simulink model "Challenge_integral"  (R2021a)
settings: Solver=VariableStepAuto  StartTime=0.0  StopTime=2.5  RelTol=1e-3
undefined symbols (not defined in the file): challint, degs2rpm, rpm2rads, sens
settings Model: Creator=gioel  LastModifiedBy=gioel

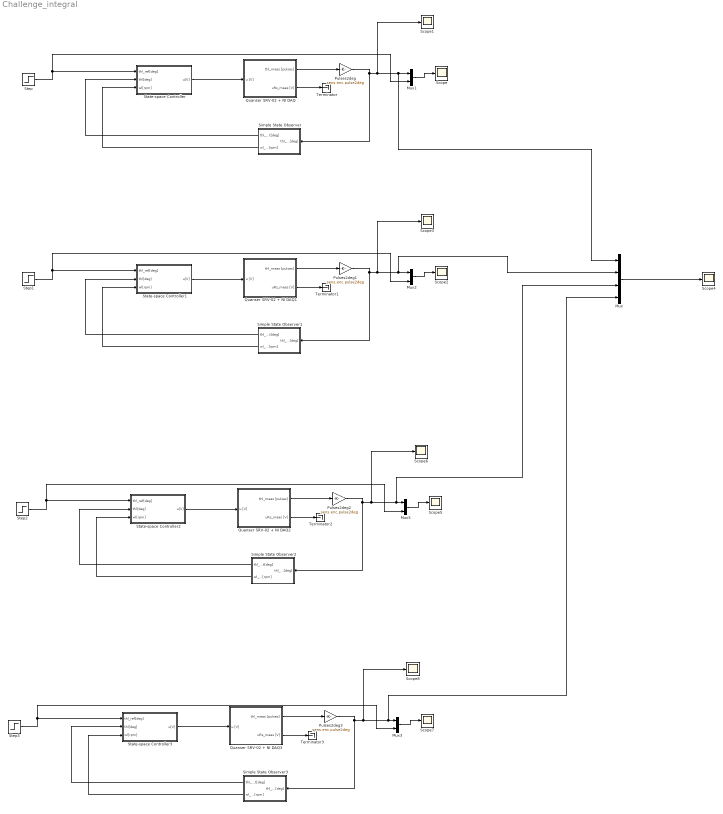
== system Challenge_integral ==
  Mux : Mux
  Mux{1..3,5} (4 alike) : Mux  Inputs=2
  Pulses2deg{,1..3} (4 alike) : Gain  Gain=sens.enc.pulse2deg
  Quanser SRV-02 + NI DAQ : Subsystem  mask(Quanser SRV-02 (with inertial load) + NI DAQ){Ts=0.001, fricType=Karnopp}
      mask prompts: Ts "NI DAQ Sample Time:"; fricType "Friction model"
      mask help: Quanser SRV-02 (with inertial load) + NI DAQ model.
      mask init:
      | %%  Sensors data
      | 
      | %   shunt resistor
      | sens.curr.Rs = 0.5;                         %   resistance [Ohm]   
      | sens.curr.uRs_std = 0.01;                   %   voltage noise standard dev [V]                           
      | sens.curr.uRs_var = sens.curr.uRs_std^2;	%   voltage noise variance [V^2]
      | 
      | %   Hewlett-Packard HEDS-5540#A06 optical encoder
      | sens.enc.ppr = 500*4;                       %   pulses per rotation
      | sens.enc.pulse2deg = 360/sens.enc.ppr;      %   [pulses] -> [deg]
      | sens.enc.pulse2rad = 2*pi/sens.enc.ppr;     %   [pulses] -> [rad]
      | sens.enc.deg2pulse = sens.enc.ppr/360;      %   [deg] -> [pulses]
      | sens.enc.rad2pulse = sens.enc.ppr/2/pi;     %   [rad] -> [pulses]
      | 
      | 
      | %%  Data acquisition board (daq) data
      | 
      | %   NI PCI-6221 DAC data
      | daq.dac.bits = 16;                                  %   resolution (bits)
      | daq.dac.fs   = 10;                                  %   full scale 
      | daq.dac.q    = 2*daq.dac.fs/(2^daq.dac.bits-1);     %	quantization
      | 
      | %   NI PCI-6221 ADC data
      | daq.adc.bits = 16;                                  %   resolution (bits)
      | daq.adc.fs   = 10;                                  %   full scale (as set in SLDRT Analog Input block)
      | daq.adc.q    = 2*daq.adc.fs/(2^daq.adc.bits-1);     %   quantization
      mask Help:
      | Riccardo Antonello (antonello@dei.unipd.it)
      | 
      | April 24, 2020
      | 
      | Dept. of Information Engineering, University of Padova
      mask TypeOptions fricType: Coulomb + viscous | Karnopp
  Quanser SRV-02 + NI DAQ1 : Subsystem  mask(Quanser SRV-02 (with inertial load) + NI DAQ){Ts=0.001, fricType=Karnopp}
      mask prompts: Ts "NI DAQ Sample Time:"; fricType "Friction model"
      mask help: Quanser SRV-02 (with inertial load) + NI DAQ model.
      mask init: same as Challenge_integral/Quanser SRV-02 + NI DAQ
      mask Help:
      | Riccardo Antonello (antonello@dei.unipd.it)
      | 
      | April 24, 2020
      | 
      | Dept. of Information Engineering, University of Padova
      mask TypeOptions fricType: Coulomb + viscous | Karnopp
  Quanser SRV-02 + NI DAQ2 : Subsystem  mask(Quanser SRV-02 (with inertial load) + NI DAQ){Ts=0.001, fricType=Karnopp}
      mask prompts: Ts "NI DAQ Sample Time:"; fricType "Friction model"
      mask help: Quanser SRV-02 (with inertial load) + NI DAQ model.
      mask init: same as Challenge_integral/Quanser SRV-02 + NI DAQ
      mask Help:
      | Riccardo Antonello (antonello@dei.unipd.it)
      | 
      | April 24, 2020
      | 
      | Dept. of Information Engineering, University of Padova
      mask TypeOptions fricType: Coulomb + viscous | Karnopp
  Quanser SRV-02 + NI DAQ3 : Subsystem  mask(Quanser SRV-02 (with inertial load) + NI DAQ){Ts=0.001, fricType=Karnopp}
      mask prompts: Ts "NI DAQ Sample Time:"; fricType "Friction model"
      mask help: Quanser SRV-02 (with inertial load) + NI DAQ model.
      mask init: same as Challenge_integral/Quanser SRV-02 + NI DAQ
      mask Help:
      | Riccardo Antonello (antonello@dei.unipd.it)
      | 
      | April 24, 2020
      | 
      | Dept. of Information Engineering, University of Padova
      mask TypeOptions fricType: Coulomb + viscous | Karnopp
  Scope{,1..8} (9 alike) : Scope
  Simple State Observer : Subsystem
  Simple State Observer1 : Subsystem
  Simple State Observer2 : Subsystem
  Simple State Observer3 : Subsystem
  State-space Controller : Subsystem
  State-space Controller1 : Subsystem
  State-space Controller2 : Subsystem
  State-space Controller3 : Subsystem
  Step{,1..3} (4 alike) : Step  Time=0  After=70  SampleTime=0
  Terminator{,1..3} (4 alike) : Terminator
  wires:
  Step/1 -> State-space Controller/1(thl_ref[deg]), Mux1/2
  Pulses2deg/1 -> Scope1/1, Mux/1, Mux1/1, Simple State Observer/1(thl_meas[deg])
  Mux1/1 -> Scope/1
  Quanser SRV-02 + NI DAQ/2(uRs_meas [V]) -> Terminator/1
  Quanser SRV-02 + NI DAQ/1(thl_meas [pulses]) -> Pulses2deg/1
  State-space Controller/1(u[V]) -> Quanser SRV-02 + NI DAQ/1(u [V])
  Simple State Observer/1(thl_est[deg]) -> State-space Controller/2(thl[deg])
  Simple State Observer/2(wl_est[rpm]) -> State-space Controller/3(wl[rpm])
  Step1/1 -> State-space Controller1/1(thl_ref[deg]), Mux2/2
  State-space Controller1/1(u[V]) -> Quanser SRV-02 + NI DAQ1/1(u [V])
  Pulses2deg1/1 -> Scope3/1, Mux/2, Mux2/1, Simple State Observer1/1(thl_meas[deg])
  Mux2/1 -> Scope2/1
  Quanser SRV-02 + NI DAQ1/2(uRs_meas [V]) -> Terminator1/1
  Simple State Observer1/2(wl_est[rpm]) -> State-space Controller1/3(wl[rpm])
  Simple State Observer1/1(thl_est[deg]) -> State-space Controller1/2(thl[deg])
  Quanser SRV-02 + NI DAQ1/1(thl_meas [pulses]) -> Pulses2deg1/1
  Step2/1 -> State-space Controller2/1(thl_ref[deg]), Mux5/2
  State-space Controller2/1(u[V]) -> Quanser SRV-02 + NI DAQ2/1(u [V])
  Pulses2deg2/1 -> Scope6/1, Mux/3, Mux5/1, Simple State Observer2/1(thl_meas[deg])
  Mux5/1 -> Scope5/1
  Quanser SRV-02 + NI DAQ2/2(uRs_meas [V]) -> Terminator2/1
  Simple State Observer2/2(wl_est[rpm]) -> State-space Controller2/3(wl[rpm])
  Simple State Observer2/1(thl_est[deg]) -> State-space Controller2/2(thl[deg])
  Quanser SRV-02 + NI DAQ2/1(thl_meas [pulses]) -> Pulses2deg2/1
  Mux/1 -> Scope4/1
  Simple State Observer3/1(thl_est[deg]) -> State-space Controller3/2(thl[deg])
  Quanser SRV-02 + NI DAQ3/2(uRs_meas [V]) -> Terminator3/1
  Simple State Observer3/2(wl_est[rpm]) -> State-space Controller3/3(wl[rpm])
  Mux3/1 -> Scope7/1
  Quanser SRV-02 + NI DAQ3/1(thl_meas [pulses]) -> Pulses2deg3/1
  Pulses2deg3/1 -> Scope8/1, Mux/4, Mux3/1, Simple State Observer3/1(thl_meas[deg])
  Step3/1 -> State-space Controller3/1(thl_ref[deg]), Mux3/2
  State-space Controller3/1(u[V]) -> Quanser SRV-02 + NI DAQ3/1(u [V])

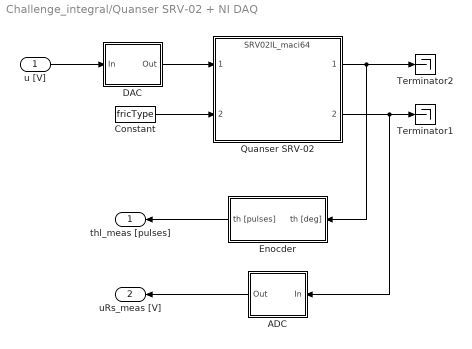
== system Challenge_integral/Quanser SRV-02 + NI DAQ ==
  u [V] : Inport
  ADC : Subsystem
  Constant : Constant  Value=fricType
  DAC : Subsystem
  Enocder : Subsystem
  Quanser SRV-02 : ModelReference  ModelNameDialog=SRV02IL_maci64.slxp  ModelReferenceVersion=1.44  CopyOfModelProtected=on
  Terminator1 : Terminator
  Terminator2 : Terminator
  thl_meas [pulses] : Outport
  uRs_meas [V] : Outport  Port=2
  wires:
  Enocder/1(th [pulses]) -> thl_meas [pulses]/1
  ADC/1(Out) -> uRs_meas [V]/1
  DAC/1(Out) -> Quanser SRV-02/1
  Quanser SRV-02/2 -> ADC/1(In), Terminator1/1
  u [V]/1 -> DAC/1(In)
  Quanser SRV-02/1 -> Enocder/1(th [deg]), Terminator2/1
  Constant/1 -> Quanser SRV-02/2

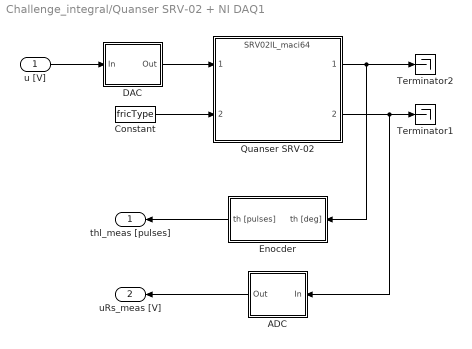
== system Challenge_integral/Quanser SRV-02 + NI DAQ1 ==
  u [V] : Inport
  ADC : Subsystem
  Constant : Constant  Value=fricType
  DAC : Subsystem
  Enocder : Subsystem
  Quanser SRV-02 : ModelReference  ModelNameDialog=SRV02IL_maci64.slxp  ModelReferenceVersion=1.44  CopyOfModelProtected=on
  Terminator1 : Terminator
  Terminator2 : Terminator
  thl_meas [pulses] : Outport
  uRs_meas [V] : Outport  Port=2
  wires:
  Enocder/1(th [pulses]) -> thl_meas [pulses]/1
  ADC/1(Out) -> uRs_meas [V]/1
  DAC/1(Out) -> Quanser SRV-02/1
  Quanser SRV-02/2 -> ADC/1(In), Terminator1/1
  u [V]/1 -> DAC/1(In)
  Quanser SRV-02/1 -> Enocder/1(th [deg]), Terminator2/1
  Constant/1 -> Quanser SRV-02/2

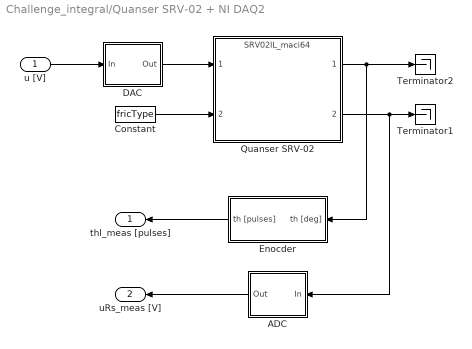
== system Challenge_integral/Quanser SRV-02 + NI DAQ2 ==
  u [V] : Inport
  ADC : Subsystem
  Constant : Constant  Value=fricType
  DAC : Subsystem
  Enocder : Subsystem
  Quanser SRV-02 : ModelReference  ModelNameDialog=SRV02IL_maci64.slxp  ModelReferenceVersion=1.44  CopyOfModelProtected=on
  Terminator1 : Terminator
  Terminator2 : Terminator
  thl_meas [pulses] : Outport
  uRs_meas [V] : Outport  Port=2
  wires:
  Enocder/1(th [pulses]) -> thl_meas [pulses]/1
  ADC/1(Out) -> uRs_meas [V]/1
  DAC/1(Out) -> Quanser SRV-02/1
  Quanser SRV-02/2 -> ADC/1(In), Terminator1/1
  u [V]/1 -> DAC/1(In)
  Quanser SRV-02/1 -> Enocder/1(th [deg]), Terminator2/1
  Constant/1 -> Quanser SRV-02/2

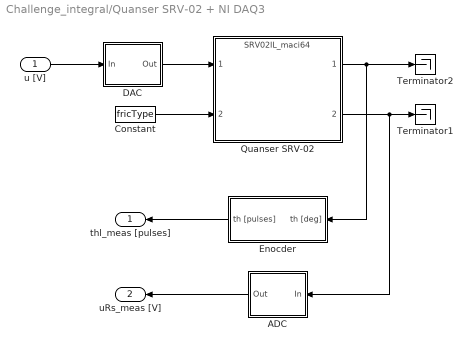
== system Challenge_integral/Quanser SRV-02 + NI DAQ3 ==
  u [V] : Inport
  ADC : Subsystem
  Constant : Constant  Value=fricType
  DAC : Subsystem
  Enocder : Subsystem
  Quanser SRV-02 : ModelReference  ModelNameDialog=SRV02IL_maci64.slxp  ModelReferenceVersion=1.44  CopyOfModelProtected=on
  Terminator1 : Terminator
  Terminator2 : Terminator
  thl_meas [pulses] : Outport
  uRs_meas [V] : Outport  Port=2
  wires:
  Enocder/1(th [pulses]) -> thl_meas [pulses]/1
  ADC/1(Out) -> uRs_meas [V]/1
  DAC/1(Out) -> Quanser SRV-02/1
  Quanser SRV-02/2 -> ADC/1(In), Terminator1/1
  u [V]/1 -> DAC/1(In)
  Quanser SRV-02/1 -> Enocder/1(th [deg]), Terminator2/1
  Constant/1 -> Quanser SRV-02/2

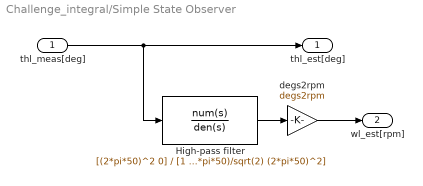
== system Challenge_integral/Simple State Observer ==
  thl_meas[deg] : Inport
  High-pass filter : TransferFcn  Numerator=[(2*pi*50)^2 0]  Denominator=[1 (2*2*pi*50)/sqrt(2) (2*pi*50)^2]
  degs2rpm : Gain  Gain=degs2rpm
  thl_est[deg] : Outport
  wl_est[rpm] : Outport  Port=2
  wires:
  High-pass filter/1 -> degs2rpm/1
  degs2rpm/1 -> wl_est[rpm]/1
  thl_meas[deg]/1 -> thl_est[deg]/1, High-pass filter/1

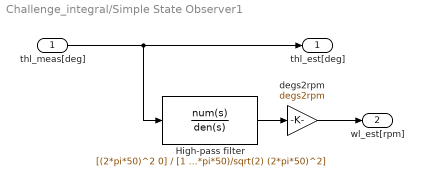
== system Challenge_integral/Simple State Observer1 ==
  thl_meas[deg] : Inport
  High-pass filter : TransferFcn  Numerator=[(2*pi*50)^2 0]  Denominator=[1 (2*2*pi*50)/sqrt(2) (2*pi*50)^2]
  degs2rpm : Gain  Gain=degs2rpm
  thl_est[deg] : Outport
  wl_est[rpm] : Outport  Port=2
  wires:
  High-pass filter/1 -> degs2rpm/1
  degs2rpm/1 -> wl_est[rpm]/1
  thl_meas[deg]/1 -> thl_est[deg]/1, High-pass filter/1

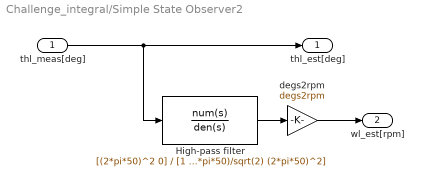
== system Challenge_integral/Simple State Observer2 ==
  thl_meas[deg] : Inport
  High-pass filter : TransferFcn  Numerator=[(2*pi*50)^2 0]  Denominator=[1 (2*2*pi*50)/sqrt(2) (2*pi*50)^2]
  degs2rpm : Gain  Gain=degs2rpm
  thl_est[deg] : Outport
  wl_est[rpm] : Outport  Port=2
  wires:
  High-pass filter/1 -> degs2rpm/1
  degs2rpm/1 -> wl_est[rpm]/1
  thl_meas[deg]/1 -> thl_est[deg]/1, High-pass filter/1

== system Challenge_integral/Simple State Observer3 ==
  thl_meas[deg] : Inport
  High-pass filter : TransferFcn  Numerator=[(2*pi*50)^2 0]  Denominator=[1 (2*2*pi*50)/sqrt(2) (2*pi*50)^2]
  degs2rpm : Gain  Gain=degs2rpm
  thl_est[deg] : Outport
  wl_est[rpm] : Outport  Port=2
  wires:
  High-pass filter/1 -> degs2rpm/1
  degs2rpm/1 -> wl_est[rpm]/1
  thl_meas[deg]/1 -> thl_est[deg]/1, High-pass filter/1

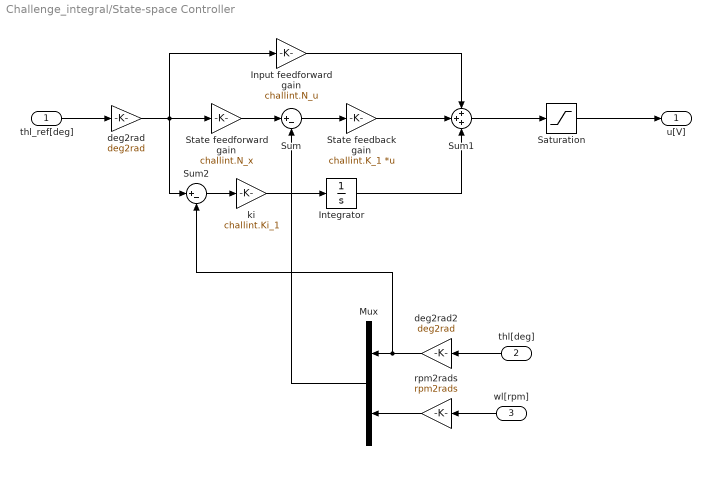
== system Challenge_integral/State-space Controller ==
  thl_ref[deg] : Inport
  thl[deg] : Inport  Port=2
  wl[rpm] : Inport  Port=3
  Input feedforward gain : Gain  Gain=challint.N_u
  Integrator : Integrator
  Mux : Mux  Inputs=2
  Saturation : Saturate  UpperLimit=10  LowerLimit=-10
  State feedback gain : Gain  Gain=challint.K_1  Multiplication=Matrix(K*u)
  State feedforward gain : Gain  Gain=challint.N_x
  Sum : Sum  Inputs=|+-
  Sum1 : Sum  Inputs=+++
  Sum2 : Sum  Inputs=|+-
  deg2rad : Gain  Gain=deg2rad
  deg2rad2 : Gain  Gain=deg2rad
  ki : Gain  Gain=challint.Ki_1
  rpm2rads : Gain  Gain=rpm2rads
  u[V] : Outport
  wires:
  rpm2rads/1 -> Mux/2
  thl_ref[deg]/1 -> deg2rad/1
  wl[rpm]/1 -> rpm2rads/1
  deg2rad/1 -> Sum2/1, Input feedforward gain/1, State feedforward gain/1
  thl[deg]/1 -> deg2rad2/1
  Saturation/1 -> u[V]/1
  State feedforward gain/1 -> Sum/1
  Sum/1 -> State feedback gain/1
  Mux/1 -> Sum/2
  Sum1/1 -> Saturation/1
  Input feedforward gain/1 -> Sum1/1
  State feedback gain/1 -> Sum1/2
  Sum2/1 -> ki/1
  deg2rad2/1 -> Sum2/2, Mux/1
  ki/1 -> Integrator/1
  Integrator/1 -> Sum1/3

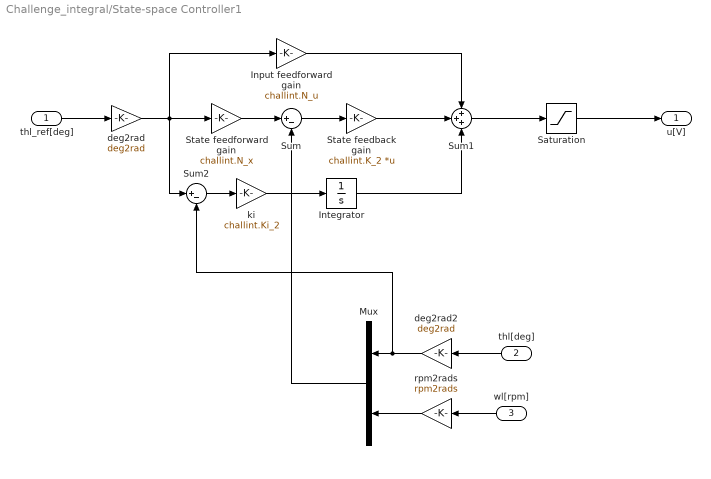
== system Challenge_integral/State-space Controller1 ==
  thl_ref[deg] : Inport
  thl[deg] : Inport  Port=2
  wl[rpm] : Inport  Port=3
  Input feedforward gain : Gain  Gain=challint.N_u
  Integrator : Integrator
  Mux : Mux  Inputs=2
  Saturation : Saturate  UpperLimit=10  LowerLimit=-10
  State feedback gain : Gain  Gain=challint.K_2  Multiplication=Matrix(K*u)
  State feedforward gain : Gain  Gain=challint.N_x
  Sum : Sum  Inputs=|+-
  Sum1 : Sum  Inputs=+++
  Sum2 : Sum  Inputs=|+-
  deg2rad : Gain  Gain=deg2rad
  deg2rad2 : Gain  Gain=deg2rad
  ki : Gain  Gain=challint.Ki_2
  rpm2rads : Gain  Gain=rpm2rads
  u[V] : Outport
  wires:
  rpm2rads/1 -> Mux/2
  thl_ref[deg]/1 -> deg2rad/1
  wl[rpm]/1 -> rpm2rads/1
  deg2rad/1 -> Sum2/1, Input feedforward gain/1, State feedforward gain/1
  thl[deg]/1 -> deg2rad2/1
  Saturation/1 -> u[V]/1
  State feedforward gain/1 -> Sum/1
  Sum/1 -> State feedback gain/1
  Mux/1 -> Sum/2
  Sum1/1 -> Saturation/1
  Input feedforward gain/1 -> Sum1/1
  State feedback gain/1 -> Sum1/2
  Sum2/1 -> ki/1
  deg2rad2/1 -> Sum2/2, Mux/1
  ki/1 -> Integrator/1
  Integrator/1 -> Sum1/3

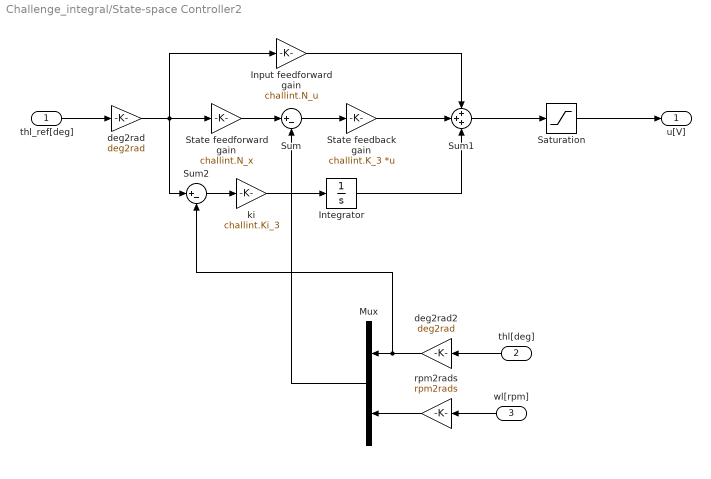
== system Challenge_integral/State-space Controller2 ==
  thl_ref[deg] : Inport
  thl[deg] : Inport  Port=2
  wl[rpm] : Inport  Port=3
  Input feedforward gain : Gain  Gain=challint.N_u
  Integrator : Integrator
  Mux : Mux  Inputs=2
  Saturation : Saturate  UpperLimit=10  LowerLimit=-10
  State feedback gain : Gain  Gain=challint.K_3  Multiplication=Matrix(K*u)
  State feedforward gain : Gain  Gain=challint.N_x
  Sum : Sum  Inputs=|+-
  Sum1 : Sum  Inputs=+++
  Sum2 : Sum  Inputs=|+-
  deg2rad : Gain  Gain=deg2rad
  deg2rad2 : Gain  Gain=deg2rad
  ki : Gain  Gain=challint.Ki_3
  rpm2rads : Gain  Gain=rpm2rads
  u[V] : Outport
  wires:
  rpm2rads/1 -> Mux/2
  thl_ref[deg]/1 -> deg2rad/1
  wl[rpm]/1 -> rpm2rads/1
  deg2rad/1 -> Sum2/1, Input feedforward gain/1, State feedforward gain/1
  thl[deg]/1 -> deg2rad2/1
  Saturation/1 -> u[V]/1
  State feedforward gain/1 -> Sum/1
  Sum/1 -> State feedback gain/1
  Mux/1 -> Sum/2
  Sum1/1 -> Saturation/1
  Input feedforward gain/1 -> Sum1/1
  State feedback gain/1 -> Sum1/2
  Sum2/1 -> ki/1
  deg2rad2/1 -> Sum2/2, Mux/1
  ki/1 -> Integrator/1
  Integrator/1 -> Sum1/3

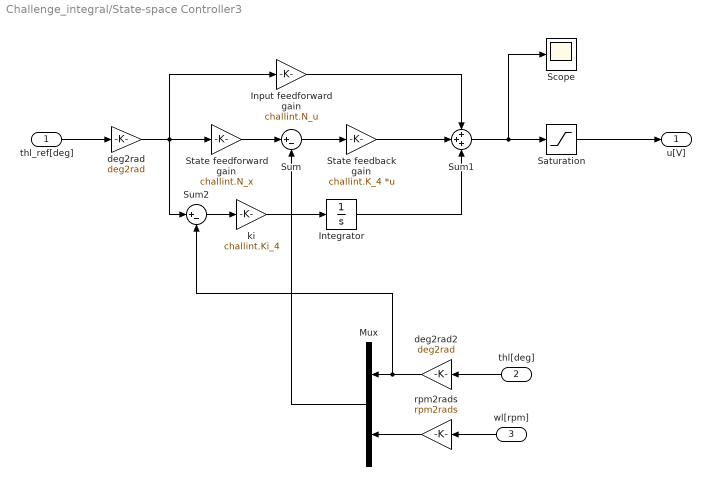
== system Challenge_integral/State-space Controller3 ==
  thl_ref[deg] : Inport
  thl[deg] : Inport  Port=2
  wl[rpm] : Inport  Port=3
  Input feedforward gain : Gain  Gain=challint.N_u
  Integrator : Integrator
  Mux : Mux  Inputs=2
  Saturation : Saturate  UpperLimit=10  LowerLimit=-10
  Scope : Scope
  State feedback gain : Gain  Gain=challint.K_4  Multiplication=Matrix(K*u)
  State feedforward gain : Gain  Gain=challint.N_x
  Sum : Sum  Inputs=|+-
  Sum1 : Sum  Inputs=+++
  Sum2 : Sum  Inputs=|+-
  deg2rad : Gain  Gain=deg2rad
  deg2rad2 : Gain  Gain=deg2rad
  ki : Gain  Gain=challint.Ki_4
  rpm2rads : Gain  Gain=rpm2rads
  u[V] : Outport
  wires:
  rpm2rads/1 -> Mux/2
  thl_ref[deg]/1 -> deg2rad/1
  wl[rpm]/1 -> rpm2rads/1
  deg2rad/1 -> Sum2/1, Input feedforward gain/1, State feedforward gain/1
  thl[deg]/1 -> deg2rad2/1
  Saturation/1 -> u[V]/1
  State feedforward gain/1 -> Sum/1
  Sum/1 -> State feedback gain/1
  Mux/1 -> Sum/2
  Sum1/1 -> Scope/1, Saturation/1
  Input feedforward gain/1 -> Sum1/1
  State feedback gain/1 -> Sum1/2
  Sum2/1 -> ki/1
  deg2rad2/1 -> Sum2/2, Mux/1
  ki/1 -> Integrator/1
  Integrator/1 -> Sum1/3

== system Challenge_integral/Quanser SRV-02 + NI DAQ/ADC ==
  In : Inport
  Quantizer : Quantizer  QuantizationInterval=daq.adc.q
  Saturation : Saturate  UpperLimit=daq.adc.fs  LowerLimit=-daq.adc.fs
  Zero-Order Hold : ZeroOrderHold  SampleTime=Ts
  Out : Outport
  wires:
  Saturation/1 -> Out/1
  In/1 -> Zero-Order Hold/1
  Quantizer/1 -> Saturation/1
  Zero-Order Hold/1 -> Quantizer/1

== system Challenge_integral/Quanser SRV-02 + NI DAQ/DAC ==
  In : Inport
  Quantizer : Quantizer  QuantizationInterval=daq.dac.q
  Saturation : Saturate  UpperLimit=daq.dac.fs  LowerLimit=-daq.dac.fs
  Zero-Order Hold : ZeroOrderHold  SampleTime=Ts
  Out : Outport
  wires:
  Quantizer/1 -> Saturation/1
  In/1 -> Zero-Order Hold/1
  Zero-Order Hold/1 -> Quantizer/1
  Saturation/1 -> Out/1

== system Challenge_integral/Quanser SRV-02 + NI DAQ/Enocder ==
  th [deg] : Inport
  Quantizer : Quantizer  QuantizationInterval=sens.enc.pulse2deg
  Zero-Order Hold : ZeroOrderHold  SampleTime=Ts
  deg2pulse : Gain  Gain=sens.enc.deg2pulse
  th [pulses] : Outport
  wires:
  Quantizer/1 -> deg2pulse/1
  th [deg]/1 -> Zero-Order Hold/1
  Zero-Order Hold/1 -> Quantizer/1
  deg2pulse/1 -> th [pulses]/1

== system Challenge_integral/Quanser SRV-02 + NI DAQ1/ADC ==
  In : Inport
  Quantizer : Quantizer  QuantizationInterval=daq.adc.q
  Saturation : Saturate  UpperLimit=daq.adc.fs  LowerLimit=-daq.adc.fs
  Zero-Order Hold : ZeroOrderHold  SampleTime=Ts
  Out : Outport
  wires:
  Saturation/1 -> Out/1
  In/1 -> Zero-Order Hold/1
  Quantizer/1 -> Saturation/1
  Zero-Order Hold/1 -> Quantizer/1

== system Challenge_integral/Quanser SRV-02 + NI DAQ1/DAC ==
  In : Inport
  Quantizer : Quantizer  QuantizationInterval=daq.dac.q
  Saturation : Saturate  UpperLimit=daq.dac.fs  LowerLimit=-daq.dac.fs
  Zero-Order Hold : ZeroOrderHold  SampleTime=Ts
  Out : Outport
  wires:
  Quantizer/1 -> Saturation/1
  In/1 -> Zero-Order Hold/1
  Zero-Order Hold/1 -> Quantizer/1
  Saturation/1 -> Out/1

== system Challenge_integral/Quanser SRV-02 + NI DAQ1/Enocder ==
  th [deg] : Inport
  Quantizer : Quantizer  QuantizationInterval=sens.enc.pulse2deg
  Zero-Order Hold : ZeroOrderHold  SampleTime=Ts
  deg2pulse : Gain  Gain=sens.enc.deg2pulse
  th [pulses] : Outport
  wires:
  Quantizer/1 -> deg2pulse/1
  th [deg]/1 -> Zero-Order Hold/1
  Zero-Order Hold/1 -> Quantizer/1
  deg2pulse/1 -> th [pulses]/1

== system Challenge_integral/Quanser SRV-02 + NI DAQ2/ADC ==
  In : Inport
  Quantizer : Quantizer  QuantizationInterval=daq.adc.q
  Saturation : Saturate  UpperLimit=daq.adc.fs  LowerLimit=-daq.adc.fs
  Zero-Order Hold : ZeroOrderHold  SampleTime=Ts
  Out : Outport
  wires:
  Saturation/1 -> Out/1
  In/1 -> Zero-Order Hold/1
  Quantizer/1 -> Saturation/1
  Zero-Order Hold/1 -> Quantizer/1

== system Challenge_integral/Quanser SRV-02 + NI DAQ2/DAC ==
  In : Inport
  Quantizer : Quantizer  QuantizationInterval=daq.dac.q
  Saturation : Saturate  UpperLimit=daq.dac.fs  LowerLimit=-daq.dac.fs
  Zero-Order Hold : ZeroOrderHold  SampleTime=Ts
  Out : Outport
  wires:
  Quantizer/1 -> Saturation/1
  In/1 -> Zero-Order Hold/1
  Zero-Order Hold/1 -> Quantizer/1
  Saturation/1 -> Out/1

== system Challenge_integral/Quanser SRV-02 + NI DAQ2/Enocder ==
  th [deg] : Inport
  Quantizer : Quantizer  QuantizationInterval=sens.enc.pulse2deg
  Zero-Order Hold : ZeroOrderHold  SampleTime=Ts
  deg2pulse : Gain  Gain=sens.enc.deg2pulse
  th [pulses] : Outport
  wires:
  Quantizer/1 -> deg2pulse/1
  th [deg]/1 -> Zero-Order Hold/1
  Zero-Order Hold/1 -> Quantizer/1
  deg2pulse/1 -> th [pulses]/1

== system Challenge_integral/Quanser SRV-02 + NI DAQ3/ADC ==
  In : Inport
  Quantizer : Quantizer  QuantizationInterval=daq.adc.q
  Saturation : Saturate  UpperLimit=daq.adc.fs  LowerLimit=-daq.adc.fs
  Zero-Order Hold : ZeroOrderHold  SampleTime=Ts
  Out : Outport
  wires:
  Saturation/1 -> Out/1
  In/1 -> Zero-Order Hold/1
  Quantizer/1 -> Saturation/1
  Zero-Order Hold/1 -> Quantizer/1

== system Challenge_integral/Quanser SRV-02 + NI DAQ3/DAC ==
  In : Inport
  Quantizer : Quantizer  QuantizationInterval=daq.dac.q
  Saturation : Saturate  UpperLimit=daq.dac.fs  LowerLimit=-daq.dac.fs
  Zero-Order Hold : ZeroOrderHold  SampleTime=Ts
  Out : Outport
  wires:
  Quantizer/1 -> Saturation/1
  In/1 -> Zero-Order Hold/1
  Zero-Order Hold/1 -> Quantizer/1
  Saturation/1 -> Out/1

== system Challenge_integral/Quanser SRV-02 + NI DAQ3/Enocder ==
  th [deg] : Inport
  Quantizer : Quantizer  QuantizationInterval=sens.enc.pulse2deg
  Zero-Order Hold : ZeroOrderHold  SampleTime=Ts
  deg2pulse : Gain  Gain=sens.enc.deg2pulse
  th [pulses] : Outport
  wires:
  Quantizer/1 -> deg2pulse/1
  th [deg]/1 -> Zero-Order Hold/1
  Zero-Order Hold/1 -> Quantizer/1
  deg2pulse/1 -> th [pulses]/1
